simulink model "Inner_Loop_NonLinear_DCM_PWM"  (R2024b)
settings: Solver=ode15s  StartTime=0.0  StopTime=0.1  RelTol=1e-6  AbsTol=1e-8
undefined symbols (not defined in the file or in its folder): bypass_inverter, Ci, converter, ctrl, DiscIntNeverNeededParam, i_start, i_stop, shaft, Tload, Ts
settings Model: SimulationMode=accelerator  Creator=rs  LastModifiedBy=overflow
settings SolverCC: AutoScaleAbsTol=off  ZeroCrossAlgorithm=Adaptive  AlgebraicLoopSolver=TrustRegion
settings DataIOCC: SaveFormat=Array  SaveOutput=off  SignalLogging=off  DSMLogging=off  SaveTime=off  ReturnWorkspaceOutputs=off  TimeSaveName=t  OutputSaveName=y
settings DebuggingCC: UnconnectedInputMsg=warning  UnconnectedOutputMsg=warning  UnconnectedLineMsg=warning  ArithmeticOperatorsInVariantConditions=warning
settings ModelReferenceCC: EnableRefExpFcnMdlSchedulingChecks=on
settings SFSimCC: SimUseLocalCustomCode=off  CustomCodeUndefinedFunction=UseInterfaceOnly
settings RTWCC: RTWUseLocalCustomCode=off  GPUComputeCapability=3.5

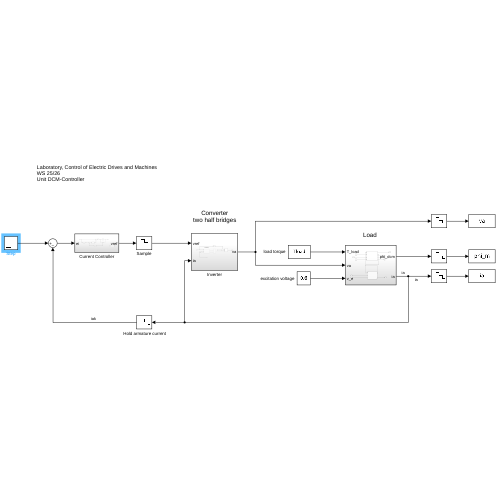
[thumbnail: Simulink's stored preview of the top-level diagram]
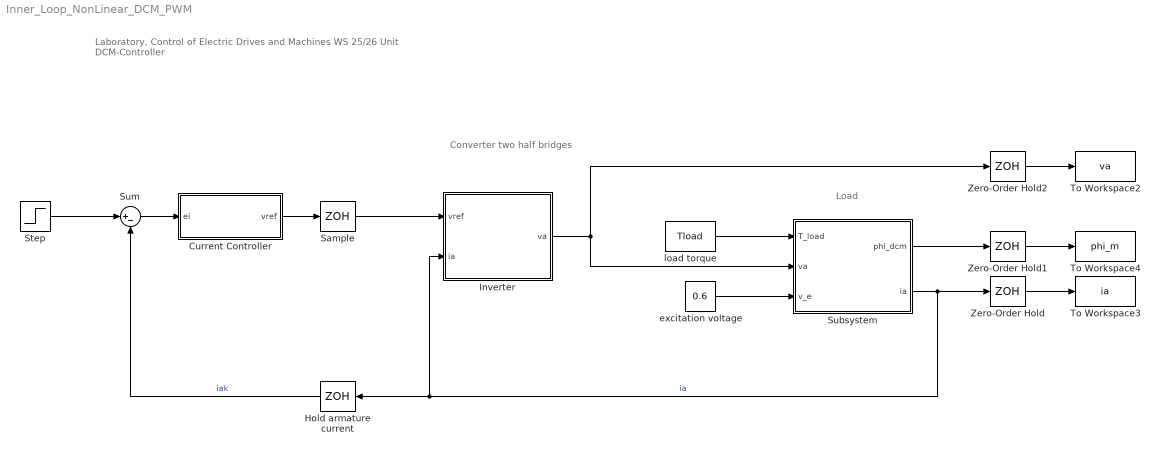
== system Inner_Loop_NonLinear_DCM_PWM ==
  note: Laboratory, Control of Electric Drives and Machines
      | WS 25/26
      | Unit DCM-Controller
  note: Load
  note: Converter
      | two half bridges
  " Hold armature current" : ZeroOrderHold  SampleTime=-1
  Current Controller : Subsystem
  Inverter : Subsystem
  Sample : ZeroOrderHold  SampleTime=-1
  Step : Step  Time=0.05  Before=i_start  After=i_stop  SampleTime=0
  Subsystem : Subsystem
  Sum : Sum  Inputs=|+-
  To Workspace2 : ToWorkspace  VariableName=va  SaveFormat=Timeseries  SampleTime=-1
  To Workspace3 : ToWorkspace  VariableName=ia  SaveFormat=Timeseries  SampleTime=-1
  To Workspace4 : ToWorkspace  VariableName=phi_m  SaveFormat=Timeseries  SampleTime=-1
  Zero-Order Hold : ZeroOrderHold  SampleTime=Ts
  Zero-Order Hold1 : ZeroOrderHold  SampleTime=Ts
  Zero-Order Hold2 : ZeroOrderHold  SampleTime=Ts
  excitation voltage : Constant  Value=0.6
  load torque : Constant  Value=Tload
  wires:
  Zero-Order Hold/1 -> To Workspace3/1
  Subsystem/2(ia) -> Inverter/2(ia), " Hold armature current"/1, Zero-Order Hold/1  "ia"
  excitation voltage/1 -> Subsystem/3(v_e)
  Zero-Order Hold2/1 -> To Workspace2/1
  Sum/1 -> Current Controller/1(ei)
  Current Controller/1(vref) -> Sample/1
  " Hold armature current"/1 -> Sum/2  "iak"
  Step/1 -> Sum/1
  Subsystem/1(phi_dcm) -> Zero-Order Hold1/1
  Inverter/1(va) -> Subsystem/2(va), Zero-Order Hold2/1
  load torque/1 -> Subsystem/1(T_load)
  Zero-Order Hold1/1 -> To Workspace4/1
  Sample/1 -> Inverter/1(vref)

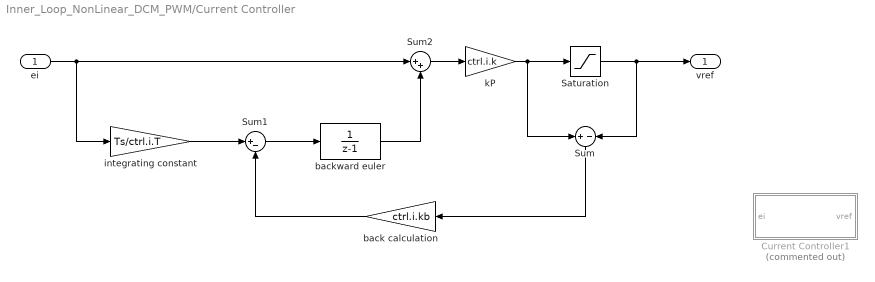
== system Inner_Loop_NonLinear_DCM_PWM/Current Controller ==
  ei : Inport
  Current Controller1 : Subsystem  Commented=on
  Saturation : Saturate  UpperLimit=ctrl.i.satP  LowerLimit=ctrl.i.satN
  Sum : Sum  Inputs=+|-
  Sum1 : Sum  Inputs=|+-
  Sum2 : Sum  Inputs=|++
  back calculation : Gain  Gain=ctrl.i.kb
  backward euler : DiscreteTransferFcn  Denominator=[1 -1]
  integrating constant : Gain  Gain=Ts/ctrl.i.T
  kP : Gain  Gain=ctrl.i.k
  vref : Outport
  wires:
  Sum1/1 -> backward euler/1
  integrating constant/1 -> Sum1/1
  Saturation/1 -> vref/1, Sum/2
  Sum/1 -> back calculation/1
  back calculation/1 -> Sum1/2
  ei/1 -> integrating constant/1, Sum2/1
  Sum2/1 -> kP/1
  kP/1 -> Sum/1, Saturation/1
  backward euler/1 -> Sum2/2

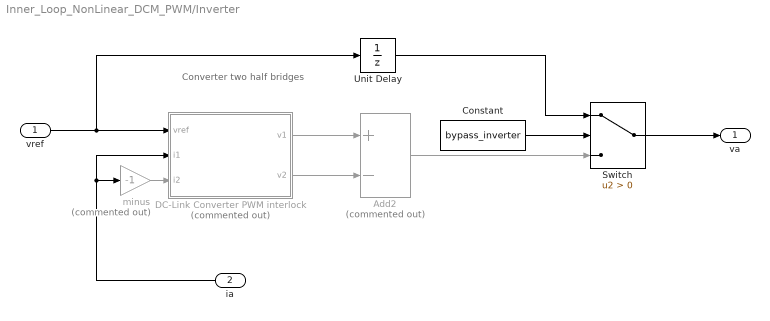
== system Inner_Loop_NonLinear_DCM_PWM/Inverter ==
  note: Converter
      | two half bridges
  vref : Inport
  ia : Inport  Port=2
  Add2 : Sum  Commented=on  Inputs=+-
  Constant : Constant  Value=bypass_inverter
  DC-Link Converter PWM interlock : Subsystem  Commented=on
  Switch : Switch  Criteria=u2 > Threshold  SaturateOnIntegerOverflow=off  InputSameDT=off
  Unit Delay : UnitDelay  SampleTime=-1  HasFrameUpgradeWarning=on
  minus : Gain  Commented=on  Gain=-1
  va : Outport
  wires:
  vref/1 -> Unit Delay/1, DC-Link Converter PWM interlock/1(vref)
  DC-Link Converter PWM interlock/2(v2) -> Add2/2
  Switch/1 -> va/1
  minus/1 -> DC-Link Converter PWM interlock/3(i2)
  Add2/1 -> Switch/3
  Constant/1 -> Switch/2
  DC-Link Converter PWM interlock/1(v1) -> Add2/1
  ia/1 -> DC-Link Converter PWM interlock/2(i1), minus/1
  Unit Delay/1 -> Switch/1

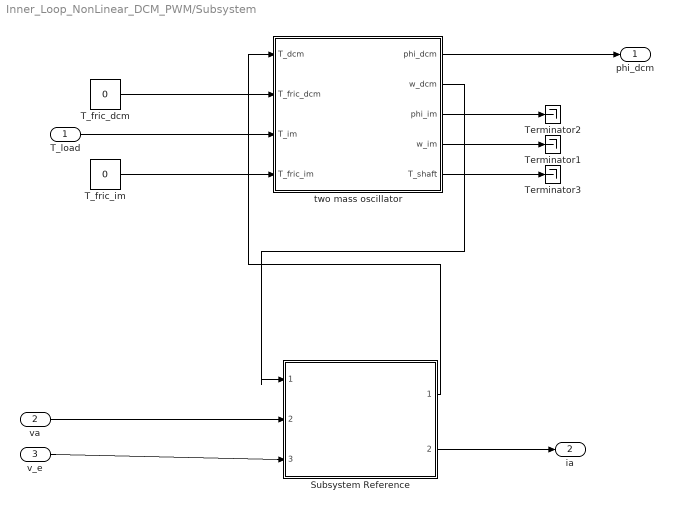
== system Inner_Loop_NonLinear_DCM_PWM/Subsystem ==
  T_load : Inport
  va : Inport  Port=2
  v_e : Inport  Port=3
  Subsystem Reference : Subsystem  ReferencedSubsystem=DCM
  T_fric_dcm : Constant  Value=0
  T_fric_im : Constant  Value=0
  Terminator1 : Terminator
  Terminator2 : Terminator
  Terminator3 : Terminator
  two mass oscillator : Subsystem
  phi_dcm : Outport
  ia : Outport  Port=2
  wires:
  two mass oscillator/5(T_shaft) -> Terminator3/1
  T_load/1 -> two mass oscillator/3(T_im)
  two mass oscillator/1(phi_dcm) -> phi_dcm/1
  two mass oscillator/4(w_im) -> Terminator1/1
  va/1 -> Subsystem Reference/2
  two mass oscillator/3(phi_im) -> Terminator2/1
  Subsystem Reference/1 -> two mass oscillator/1(T_dcm)
  two mass oscillator/2(w_dcm) -> Subsystem Reference/1
  T_fric_dcm/1 -> two mass oscillator/2(T_fric_dcm)
  T_fric_im/1 -> two mass oscillator/4(T_fric_im)
  Subsystem Reference/2 -> ia/1
  v_e/1 -> Subsystem Reference/3

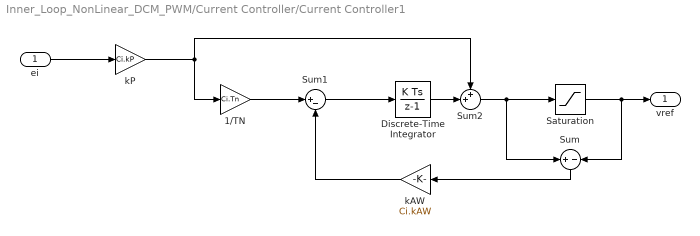
== system Inner_Loop_NonLinear_DCM_PWM/Current Controller/Current Controller1 ==
  ei : Inport
  1/TN : Gain  Gain=Ci.Tn
  Discrete-Time Integrator : DiscreteIntegrator  SampleTime=-1  ICPrevOutput=DiscIntNeverNeededParam  ICPrevScaledInput=DiscIntNeverNeededParam
  Saturation : Saturate
  Sum : Sum  Inputs=+|-
  Sum1 : Sum  Inputs=|+-
  Sum2 : Sum  Inputs=++|
  kAW : Gain  Gain=Ci.kAW
  kP : Gain  Gain=Ci.kP
  vref : Outport
  wires:
  Sum1/1 -> Discrete-Time Integrator/1
  1/TN/1 -> Sum1/1
  Discrete-Time Integrator/1 -> Sum2/2
  ei/1 -> kP/1
  Sum2/1 -> Sum/1, Saturation/1
  Saturation/1 -> Sum/2, vref/1
  Sum/1 -> kAW/1
  kAW/1 -> Sum1/2
  kP/1 -> Sum2/1, 1/TN/1

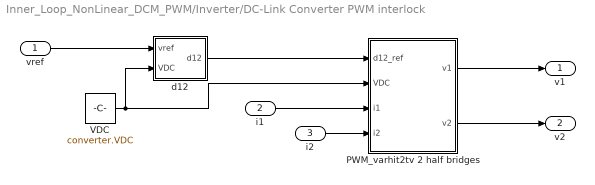
== system Inner_Loop_NonLinear_DCM_PWM/Inverter/DC-Link Converter PWM interlock ==
  vref : Inport
  i1 : Inport  Port=2
  i2 : Inport  Port=3
  PWM_varhit2tv 2 half bridges : Subsystem
  VDC : Constant  Value=converter.VDC
  d12 : Subsystem
  v1 : Outport  VectorParamsAs1DForOutWhenUnconnected=off
  v2 : Outport  Port=2  VectorParamsAs1DForOutWhenUnconnected=off
  wires:
  PWM_varhit2tv 2 half bridges/2(v2) -> v2/1
  VDC/1 -> PWM_varhit2tv 2 half bridges/2(VDC), d12/2(VDC)
  i2/1 -> PWM_varhit2tv 2 half bridges/4(i2)
  PWM_varhit2tv 2 half bridges/1(v1) -> v1/1
  d12/1(d12) -> PWM_varhit2tv 2 half bridges/1(d12_ref)
  vref/1 -> d12/1(vref)
  i1/1 -> PWM_varhit2tv 2 half bridges/3(i1)

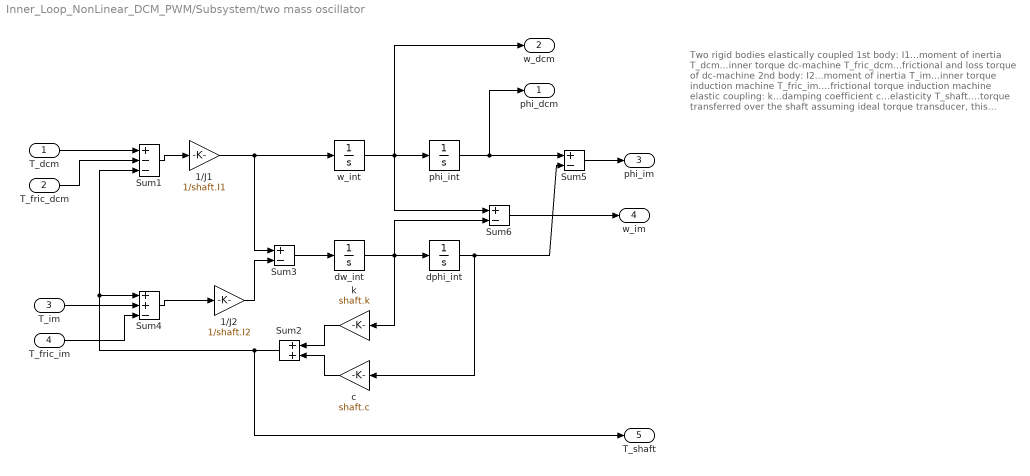
== system Inner_Loop_NonLinear_DCM_PWM/Subsystem/two mass oscillator ==
  note: Two rigid bodies elastically coupled
      |
      | 1st body:
      | I1...moment of inertia
      | T_dcm...inner torque dc-machine
      | T_fric_dcm...frictional and loss torque of dc-machine
      |
      | 2nd body:
      | I2...moment of inertia
      | T_im...inner torque induction machine
      | T_fric_im....frictional torque induction machine
      |
      | elastic coupling:
      | k...damping coefficient
      | c...elasticity
      |
      | T_shaft....torque transferred over the shaft
      |                 assuming ideal torque transducer, this equals
      |                 measured torque
      |
      | states:
      | w_dcm...angular speed of first body
      | phi_dcm...rotor position of first body
      |
      | dw....angular speed, difference w_dcm-w_im
      | dphi...position difference phi_dcm-phi_im
      |
      | incremental encoder is mounted on dc-machine side
  T_dcm : Inport
  T_fric_dcm : Inport  Port=2
  T_im : Inport  Port=3
  T_fric_im : Inport  Port=4
  1/J1 : Gain  Gain=1/shaft.I1  SaturateOnIntegerOverflow=on  OutDataTypeStr=Inherit: Same as input  ParamDataTypeStr=Inherit: Same as input
  1/J2 : Gain  Gain=1/shaft.I2  SaturateOnIntegerOverflow=on  OutDataTypeStr=Inherit: Same as input  ParamDataTypeStr=Inherit: Same as input
  Sum1 : Sum  Inputs=+--  SaturateOnIntegerOverflow=on
  Sum2 : Sum  SaturateOnIntegerOverflow=on
  Sum3 : Sum  Inputs=+-  SaturateOnIntegerOverflow=on
  Sum4 : Sum  Inputs=++-  SaturateOnIntegerOverflow=on
  Sum5 : Sum  Inputs=+-  SaturateOnIntegerOverflow=on
  Sum6 : Sum  Inputs=+-  SaturateOnIntegerOverflow=on
  c : Gain  Gain=shaft.c  SaturateOnIntegerOverflow=on  OutDataTypeStr=Inherit: Same as input  ParamDataTypeStr=Inherit: Same as input
  dphi_int : Integrator  InitialCondition=shaft.dphi_0
  dw_int : Integrator  InitialCondition=shaft.dw_0
  k : Gain  Gain=shaft.k  SaturateOnIntegerOverflow=on  OutDataTypeStr=Inherit: Same as input  ParamDataTypeStr=Inherit: Same as input
  phi_int : Integrator  InitialCondition=shaft.phi1_0
  w_int : Integrator  InitialCondition=shaft.w1_0
  phi_dcm : Outport  VectorParamsAs1DForOutWhenUnconnected=off
  w_dcm : Outport  Port=2  VectorParamsAs1DForOutWhenUnconnected=off
  phi_im : Outport  Port=3  VectorParamsAs1DForOutWhenUnconnected=off
  w_im : Outport  Port=4  VectorParamsAs1DForOutWhenUnconnected=off
  T_shaft : Outport  Port=5  VectorParamsAs1DForOutWhenUnconnected=off
  wires:
  w_int/1 -> phi_int/1, Sum6/1, w_dcm/1
  dw_int/1 -> dphi_int/1, k/1, Sum6/2
  dphi_int/1 -> c/1, Sum5/2
  k/1 -> Sum2/1
  c/1 -> Sum2/2
  Sum1/1 -> 1/J1/1
  1/J1/1 -> w_int/1, Sum3/1
  Sum3/1 -> dw_int/1
  Sum4/1 -> 1/J2/1
  1/J2/1 -> Sum3/2
  Sum2/1 -> T_shaft/1, Sum4/1, Sum1/3
  phi_int/1 -> Sum5/1, phi_dcm/1
  T_dcm/1 -> Sum1/1
  T_im/1 -> Sum4/2
  Sum5/1 -> phi_im/1
  Sum6/1 -> w_im/1
  T_fric_dcm/1 -> Sum1/2
  T_fric_im/1 -> Sum4/3

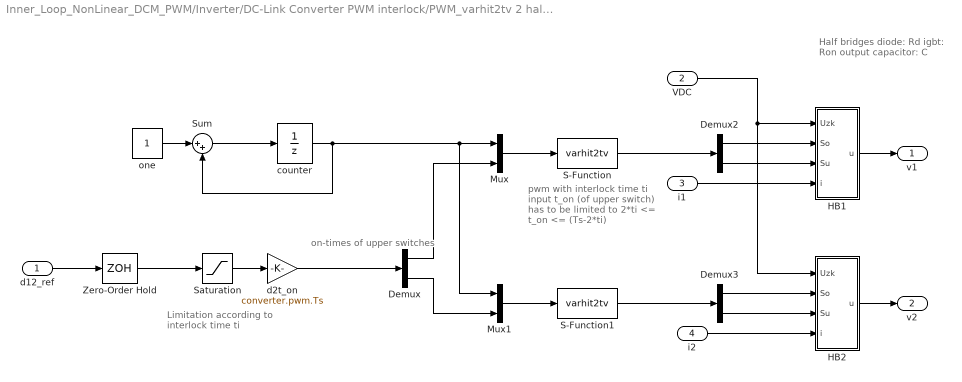
== system Inner_Loop_NonLinear_DCM_PWM/Inverter/DC-Link Converter PWM interlock/PWM_varhit2tv 2 half bridges ==
  note: on-times
      | of upper switches
  note: pwm with interlock time ti
      | input t_on (of upper switch)
      | has to be limited to
      | 2*ti <= t_on <= (Ts-2*ti)
  note: Half bridges
      | diode: Rd
      | igbt: Ron
      | output capacitor: C
  note: Limitation according to
      | interlock time ti
  d12_ref : Inport
  VDC : Inport  Port=2
  i1 : Inport  Port=3
  i2 : Inport  Port=4
  Demux : Demux  Outputs=2
  Demux2 : Demux  Outputs=2
  Demux3 : Demux  Outputs=2
  HB1 : Subsystem  mask{HB=converter.HB1}
  HB2 : Subsystem  mask{HB=converter.HB2}
  Mux : Mux  Inputs=2
  Mux1 : Mux  Inputs=2
  S-Function : S-Function  FunctionName=varhit2tv  Parameters=converter.pwm.Ts, converter.pwm.ti  SFunctionDeploymentMode=off  EnableBusSupport=off
  S-Function1 : S-Function  FunctionName=varhit2tv  Parameters=converter.pwm.Ts, converter.pwm.ti  SFunctionDeploymentMode=off  EnableBusSupport=off
  Saturation : Saturate  UpperLimit=converter.pwm.dmax  LowerLimit=converter.pwm.dmin
  Sum : Sum  Inputs=|++  SaturateOnIntegerOverflow=on
  Zero-Order Hold : ZeroOrderHold  SampleTime=converter.pwm.Ts
  counter : UnitDelay  SampleTime=[converter.pwm.Ts 0]  HasFrameUpgradeWarning=on
  d2t_on : Gain  Gain=converter.pwm.Ts  SaturateOnIntegerOverflow=on  OutDataTypeStr=Inherit: Same as input  ParamDataTypeStr=Inherit: Same as input
  one : Constant
  v1 : Outport  VectorParamsAs1DForOutWhenUnconnected=off
  v2 : Outport  Port=2  VectorParamsAs1DForOutWhenUnconnected=off
  wires:
  Sum/1 -> counter/1
  one/1 -> Sum/1
  counter/1 -> Sum/2, Mux1/1, Mux/1
  Mux/1 -> S-Function/1
  Saturation/1 -> d2t_on/1
  d12_ref/1 -> Zero-Order Hold/1
  S-Function/1 -> Demux2/1
  Mux1/1 -> S-Function1/1
  d2t_on/1 -> Demux/1
  Demux/1 -> Mux/2
  Demux/2 -> Mux1/2
  i1/1 -> HB1/4(i)
  S-Function1/1 -> Demux3/1
  Demux2/1 -> HB1/2(So)
  Demux2/2 -> HB1/3(Su)
  Demux3/1 -> HB2/2(So)
  Demux3/2 -> HB2/3(Su)
  VDC/1 -> HB2/1(Uzk), HB1/1(Uzk)
  Zero-Order Hold/1 -> Saturation/1
  HB1/1(u) -> v1/1
  HB2/1(u) -> v2/1
  i2/1 -> HB2/4(i)

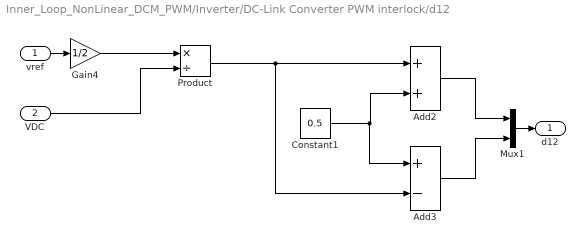
== system Inner_Loop_NonLinear_DCM_PWM/Inverter/DC-Link Converter PWM interlock/d12 ==
  vref : Inport
  VDC : Inport  Port=2
  Add2 : Sum
  Add3 : Sum  Inputs=+-
  Constant1 : Constant  Value=0.5
  Gain4 : Gain  Gain=1/2
  Mux1 : Mux  Inputs=2
  Product : Product  Inputs=*/
  d12 : Outport  VectorParamsAs1DForOutWhenUnconnected=off
  wires:
  Constant1/1 -> Add3/1, Add2/2
  Add2/1 -> Mux1/1
  Add3/1 -> Mux1/2
  Mux1/1 -> d12/1
  vref/1 -> Gain4/1
  Product/1 -> Add3/2, Add2/1
  Gain4/1 -> Product/1
  VDC/1 -> Product/2

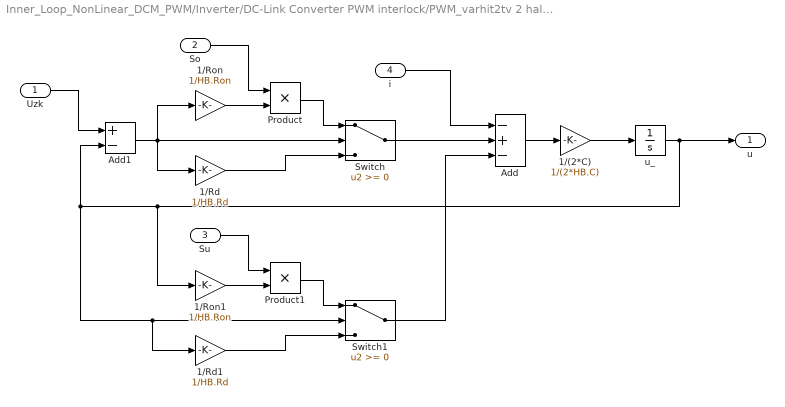
== system Inner_Loop_NonLinear_DCM_PWM/Inverter/DC-Link Converter PWM interlock/PWM_varhit2tv 2 half bridges/HB1 ==
  Uzk : Inport
  So : Inport  Port=2
  Su : Inport  Port=3
  i : Inport  Port=4
  1/(2*C) : Gain  Gain=1/(2*HB.C)
  1/Rd : Gain  Gain=1/HB.Rd
  1/Rd1 : Gain  Gain=1/HB.Rd
  1/Ron : Gain  Gain=1/HB.Ron
  1/Ron1 : Gain  Gain=1/HB.Ron
  Add : Sum  Inputs=-+-
  Add1 : Sum  Inputs=+-
  Product : Product
  Product1 : Product
  Switch : Switch  SaturateOnIntegerOverflow=off  InputSameDT=off
  Switch1 : Switch  SaturateOnIntegerOverflow=off  InputSameDT=off
  u_ : Integrator  InitialCondition=HB.u0
  u : Outport  VectorParamsAs1DForOutWhenUnconnected=off
  wires:
  Add/1 -> 1/(2*C)/1
  Switch/1 -> Add/2
  Add1/1 -> 1/Rd/1, Switch/2, 1/Ron/1
  1/Ron/1 -> Product/2
  1/(2*C)/1 -> u_/1
  1/Ron1/1 -> Product1/2
  Product1/1 -> Switch1/1
  u_/1 -> u/1, 1/Ron1/1, 1/Rd1/1, Switch1/2, Add1/2
  Switch1/1 -> Add/3
  Su/1 -> Product1/1
  i/1 -> Add/1
  1/Rd1/1 -> Switch1/3
  So/1 -> Product/1
  1/Rd/1 -> Switch/3
  Uzk/1 -> Add1/1
  Product/1 -> Switch/1

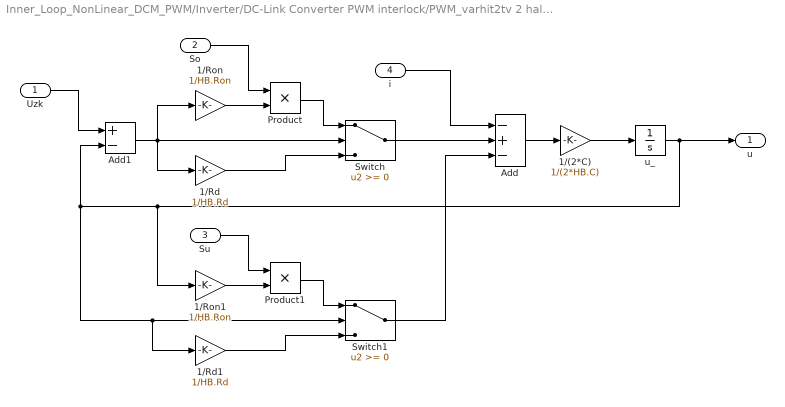
== system Inner_Loop_NonLinear_DCM_PWM/Inverter/DC-Link Converter PWM interlock/PWM_varhit2tv 2 half bridges/HB2 ==
  Uzk : Inport
  So : Inport  Port=2
  Su : Inport  Port=3
  i : Inport  Port=4
  1/(2*C) : Gain  Gain=1/(2*HB.C)
  1/Rd : Gain  Gain=1/HB.Rd
  1/Rd1 : Gain  Gain=1/HB.Rd
  1/Ron : Gain  Gain=1/HB.Ron
  1/Ron1 : Gain  Gain=1/HB.Ron
  Add : Sum  Inputs=-+-
  Add1 : Sum  Inputs=+-
  Product : Product
  Product1 : Product
  Switch : Switch  SaturateOnIntegerOverflow=off  InputSameDT=off
  Switch1 : Switch  SaturateOnIntegerOverflow=off  InputSameDT=off
  u_ : Integrator  InitialCondition=HB.u0
  u : Outport  VectorParamsAs1DForOutWhenUnconnected=off
  wires:
  Product/1 -> Switch/1
  Uzk/1 -> Add1/1
  1/Rd/1 -> Switch/3
  So/1 -> Product/1
  1/Rd1/1 -> Switch1/3
  i/1 -> Add/1
  Su/1 -> Product1/1
  Switch1/1 -> Add/3
  u_/1 -> Add1/2, Switch1/2, 1/Rd1/1, 1/Ron1/1, u/1
  Product1/1 -> Switch1/1
  1/Ron1/1 -> Product1/2
  1/(2*C)/1 -> u_/1
  1/Ron/1 -> Product/2
  Add1/1 -> 1/Ron/1, Switch/2, 1/Rd/1
  Switch/1 -> Add/2
  Add/1 -> 1/(2*C)/1
